simulink model "AirManagementSystem"  (R2018b)
settings: Solver=ode4  StartTime=0.0  StopTime=14400  FixedStep=dt  RelTol=1e-3
values from neighbouring files (symbols this model uses):
  AirSourceMode = 2    [run_sim.m]
  dt = 0.01    [run_sim.m]    (also in sys_id_pipeline.m = mean(diff(Time_vec_full)))
  K31 = Result31.K_slope    [sys_id_pipeline.m]
  K32 = Result32.K_slope    [sys_id_pipeline.m]
  P_ref = GlobalParams.P_ref    [sys_id_pipeline.m]
  Patm = GlobalParams.Patm    [sys_id_pipeline.m]
  R_gas = GlobalParams.R    [sys_id_pipeline.m]
  T_ref = GlobalParams.T_ref    [sys_id_pipeline.m]
  Tau31 = 5    [sys_id_pipeline.m]
  Tau32 = 5    [sys_id_pipeline.m]
  Tp31 = Result31.Tp    [sys_id_pipeline.m]
  Tp32 = Result32.Tp    [sys_id_pipeline.m]
  V_vol = pi * (0.05)^2 * 5    (= 0.0392699081699)    [run_sim.m]
  X31_den = sys_X31.Denominator    [sys_id_value.m]
  X31_num = sys_X31.Numerator    [sys_id_value.m]
  X32_den = sys_X32.Denominator    [sys_id_value.m]
  X32_num = sys_X32.Numerator    [sys_id_value.m]
libraries: simulink x8
(part 2 of 2)

== matlab function AirManagementSystem/ECS Controller/Smith_MPC_Controller/Smith_MPC_Controller ==
  settings: updateMethod=DISCRETE
  data: Q31Ref input; V31 output; Q31Real input; Q32Ref input; Q32Real input; P30 input; T30 input; V32 output; K31 parameter; Tau31 parameter; K32 parameter; Tau32 parameter; P_ref parameter; T_ref parameter; R_gas parameter; Patm parameter; Tp31 parameter; Tp32 parameter; dt parameter; X31_num parameter; X31_den parameter; X32_num parameter; X32_den parameter
function [V31, V32] = Smith_MPC_Controller(Q31Ref, Q31Real, Q32Ref, Q32Real, P30, T30, K31, Tau31, K32, Tau32, P_ref, T_ref, R_gas, Patm, Tp31, Tp32, dt, X31_num, X31_den, X32_num, X32_den)
    % Smith_MPC_Controller
    %
    % 这是一个基于 Smith 预估器的 MPC 控制器，用于替换原有的 Smith-PI 方案。
    % 核心思想：
    % 1. Smith 预估器：利用内部模型消除反馈回路中的纯滞后，使 MPC 面对一个"无滞后"的虚拟对象。
    % 2. MPC 控制：利用过程模型预测未来轨迹，在处理约束(0-100%)的前提下最小化跟踪误差。
    % 3. 测量滞后补偿：通过比较实际测量值与延时模型输出，估算当前扰动并修正 MPC 的状态估计。
    %
    % 适用性：
    % - Q31 (过阻尼): MPC 通过预测未来，能更果断地给出控制量，克服大惯性。
    % - Q32 (欠阻尼): MPC 的代价函数包含控制增量惩罚 (R_weight)，能有效抑制震荡。

    % === 1. 状态记忆区 ===
    persistent model_31 model_32            % 快速模型状态 [x1; x2; x3]
    persistent delay_buffer_31 delay_buffer_32 % 延时缓冲区
    persistent head_31 head_32              % 缓冲区指针
    persistent u_prev_31 u_prev_32          % 上一时刻控制量
    persistent first_run                    % 初始化标志
    
    MAX_BUF = 1000;

    if isempty(first_run)
        model_31 = [0;0;0]; model_32 = [0;0;0];
        delay_buffer_31 = zeros(MAX_BUF, 1);
        delay_buffer_32 = zeros(MAX_BUF, 1);
        head_31 = 1; head_32 = 1;
        u_prev_31 = 0; u_prev_32 = 0;
        first_run = 0;
    end

    % === 2. 全局参数与 MPC 配置 ===
    % 计算流量工况系数 (增益调度)
    Ratio = CalculateFlowRatio(P30, T30, P_ref, T_ref, R_gas, Patm);

    % MPC 调参指南：
    % N_p (预测时域): 看得越远越稳，但计算量大。过阻尼系统需要较长 N_p。
    % N_c (控制时域): 自由度。通常取 N_p 的 10%-20%。
    % lambda (控制权重): 越大系统越柔和（抗震荡），越小响应越快（抗惯性）。
    
    % --- 通道 31 配置 (过阻尼) ---
    % 策略：较小的 lambda 允许较大的动作来克服惯性/摩擦
    MPC_31.Np = 200;        % 预测 15 步
    MPC_31.Nc = 40;         % 控制 3 步变化
    MPC_31.lambda = 5;   % 权重较小，追求快速响应
    
    % --- 通道 32 配置 (欠阻尼) ---
    % 策略：较大的 lambda 抑制控制量的剧烈变化，防止激发震荡
    MPC_32.Np = 200;        % 预测更远，捕捉震荡趋势
    MPC_32.Nc = 40; 
    MPC_32.lambda = 50;   % 权重较大，强行增加阻尼效果

    % ==========================================================
    %       通道 31 控制回路 (MPC + Smith)
    % ==========================================================
    
    % 1. 获取离散化状态空间模型 (A, B, C)
    % 注意：将 Ratio 应用于 B 矩阵，使模型增益匹配当前物理工况
    [A31, B31, C31] = GetStateSpace(X31_num, X31_den, K31, Ratio, Tp31, dt);
    
    % 2. Smith 快速模型更新 (无滞后估计)
    % 计算假如没有滞后，当前系统应该在哪
    [model_31, Y_fast_31] = UpdateStateModel(model_31, u_prev_31, A31, B31, C31);
    
    % 3. 延时模型更新 (历史数据回放)
    [delay_buffer_31, head_31, Y_delayed_31] = UpdateDelayBuffer(delay_buffer_31, head_31, Y_fast_31, Tau31, dt, MAX_BUF);
    
    % 4. 测量滞后补偿 / 扰动估算
    % 真实值与模型值的差异，被认为是"扰动"(dist_est)
    dist_est_31 = Q31Real - Y_delayed_31;
    
    % 5. 构造 MPC 反馈状态
    % 修正后的输出 = 无滞后模型值 + 当前扰动
    % MPC 认为它在控制这个"当前"值，从而忽略了滞后
    y_feedback_31 = Y_fast_31 + dist_est_31;
    
    % 6. MPC 求解
    % 计算最优控制增量 du
    du_31 = SolveMPC(A31, B31, C31, MPC_31, model_31, y_feedback_31, Q31Ref, u_prev_31);
    
    % 7. 输出计算与限幅
    u_raw_31 = u_prev_31 + du_31;
    u_raw_31 = max(0, min(100, u_raw_31));
    
    % 8. (可选) 保留死区补偿作为最后一道防线
    % MPC 虽然能处理部分非线性，但物理阀门的静摩擦最好显式补偿
    V31 = InverseDeadzoneComp(u_raw_31, u_prev_31, 1.4, Q31Ref - y_feedback_31);
    u_prev_31 = V31;

    % ==========================================================
    %       通道 32 控制回路 (MPC + Smith)
    % ==========================================================
    
    [A32, B32, C32] = GetStateSpace(X32_num, X32_den, K32, Ratio, Tp32, dt);
    
    [model_32, Y_fast_32] = UpdateStateModel(model_32, u_prev_32, A32, B32, C32);
    [delay_buffer_32, head_32, Y_delayed_32] = UpdateDelayBuffer(delay_buffer_32, head_32, Y_fast_32, Tau32, dt, MAX_BUF);
    
    dist_est_32 = Q32Real - Y_delayed_32;
    y_feedback_32 = Y_fast_32 + dist_est_32;
    
    du_32 = SolveMPC(A32, B32, C32, MPC_32, model_32, y_feedback_32, Q32Ref, u_prev_32);
    
    u_raw_32 = u_prev_32 + du_32;
    u_raw_32 = max(0, min(100, u_raw_32));
    
    V32 = InverseDeadzoneComp(u_raw_32, u_prev_32, 0.5, Q32Ref - y_feedback_32);
    u_prev_32 = V32;

end

%% === 核心模块: MPC 求解器 (解析解法) ===
% 这是一个轻量级的无约束 MPC 求解器，通过饱和截断处理约束。
% 求解目标函数: J = sum((Y - Ref)^2) + lambda * sum(dU^2)
function du_opt = SolveMPC(A, B, C, Config, x_current, y_corrected, Ref, u_last)
    Np = Config.Np;
    Nc = Config.Nc;
    lambda = Config.lambda;
    
    % 1. 预计算预测矩阵 (Phi 和 Gamma)
    % Y = Phi * x0 + Gamma * dU
    % 注意：为了效率，这些矩阵在定常系统中可以离线计算。
    % 但由于我们有 Ratio 增益调度，B 矩阵是变的，所以必须实时计算。
    
    n = size(A, 1); % 状态维数
    Phi = zeros(Np, n);
    Gamma = zeros(Np, Nc);
    
    % 构建 Phi (自由响应部分)
    A_pow = eye(n);
    for i = 1:Np
        A_pow = A_pow * A;
        Phi(i, :) = C * A_pow;
    end
    
    % 构建 Gamma (受迫响应部分)
    % 这是一个下三角Toeplitz矩阵的变体，处理控制增量
    % 这种 formulation 基于 dU 模型 (积分型 MPC)，本身具有无静差特性
    
    % 这里的状态空间是基于物理状态 x 的。为了实现无静差，
    % 我们通常使用增量式 MPC 形式，或者在外部处理扰动（我们已经通过 Smith 做了）。
    % 在 Smith 架构下，我们只要让 y 追踪 Ref 即可。
    % 这里简化处理：假设 dU 在 Nc 步后为 0。
    
    % 临时计算阶跃响应系数 h
    h = zeros(Np, 1);
    AB_pow = B;
    for i = 1:Np
        h(i) = C * AB_pow;
        AB_pow = A * AB_pow + B; % 累积效果 (如果是位置式)
        % 修正：对于常规状态空间 x(k+1) = Ax + Bu, 
        % 阶跃响应 h(i) = C * (sum(A^(j-1)*B))
    end
    
    % 由于直接构造增量形式较复杂，这里采用简化的 DMC (Dynamic Matrix Control) 思路
    % 利用上面计算的阶跃响应 h 来填充 Gamma
    % Gamma 矩阵:
    % [h1   0    0 ]
    % [h2   h1   0 ]
    % [h3   h2   h1]
    
    % 重新计算阶跃响应序列 (Step Response)
    step_resp = zeros(Np, 1);
    x_tmp = zeros(n, 1);
    u_step = 1;
    for i = 1:Np
        x_tmp = A * x_tmp + B * u_step;
        step_resp(i) = C * x_tmp;
    end
    
    for i = 1:Np
        for j = 1:Nc
            if (i >= j)
                Gamma(i, j) = step_resp(i - j + 1);
            end
        end
    end
    
    % 2. 预测当前的自由响应 (Free Response)
    % 也就是假设未来 dU 全为 0，系统会怎么走
    % 这里的起点是 x_current。但在 Smith 结构中，我们有测量修正。
    % 修正量 = y_corrected - (C * x_current)
    % 我们把这个常数偏差加到自由响应上。
    
    dist = y_corrected - (C * x_current);
    
    % 自由响应预测
    Y_free = zeros(Np, 1);
    x_pred = x_current;
    u_curr = u_last; % 假设控制量保持不变
    for i = 1:Np
        x_pred = A * x_pred + B * u_curr;
        Y_free(i) = C * x_pred + dist; % 加上扰动估计
    end
    
    % 3. 构造误差向量
    E = Ref * ones(Np, 1) - Y_free;
    
    % 4. 求解最优 dU
    % 解析解: dU = (Gamma' * Gamma + lambda * I)^-1 * Gamma' * E
    H = Gamma' * Gamma + lambda * eye(Nc);
    f = -Gamma' * E;
    
    % 如果矩阵很小(Nc=3)，直接求逆很快
    dU_seq = -H \ f;
    
    % 取第一个控制增量
    du_opt = dU_seq(1);
    
    % 简单的饱和处理 (防积分饱和的一种形式)
    % 检查应用 du_opt 后是否超出 0-100
    if (u_last + du_opt) > 100
        du_opt = 100 - u_last;
    elseif (u_last + du_opt) < 0
        du_opt = 0 - u_last;
    end
end

%% === 辅助模块: 模型转换 ===
% 将传递函数参数转换为离散状态空间 A, B, C
function [A, B, C] = GetStateSpace(num, den, K, Ratio, Tp, Ts)
    % 阀门二阶: num / (s^2 + den(2)s + den(3)) -> 实际上 den 可能是 [1 2*zw*wn wn^2]
    % 这里沿用原代码逻辑：acc = K_valve * u - zw * x2 - wn2 * x1
    % 原代码系数映射: wn2 = den(3), zw = den(2), K_valve = num
    
    wn2 = den(3);
    zw = den(2);
    K_valve = num;
    K_total = K * Ratio; % 增益调度
    
    % 连续时间矩阵 (Ac, Bc)
    % 状态: [x1(阀位), x2(阀速), x3(流量)]
    % dx1 = x2
    % dx2 = -wn2*x1 - zw*x2 + K_valve*u
    % dx3 = (K_total*x1 - x3)/Tp
    
    % 离散化 (Euler 近似，与原代码一致，保持物理意义)
    % x1(k+1) = x1(k) + Ts*x2(k)
    % x2(k+1) = x2(k) - Ts*wn2*x1(k) - Ts*zw*x2(k) + Ts*K_valve*u(k)
    % x3(k+1) = x3(k) + (Ts*K_total/Tp)*x1(k) - (Ts/Tp)*x3(k)
    
    Tp = max(Tp, 0.1); % 保护
    
    A = [1,          Ts,               0;
         -Ts*wn2,    1 - Ts*zw,        0;
         Ts*K_total/Tp, 0,             1 - Ts/Tp];
         
    B = [0;
         Ts * K_valve;
         0];
         
    C = [0, 0, 1];
end

%% === 辅助模块: 模型状态更新 ===
function [state_new, y_out] = UpdateStateModel(state, u, A, B, C)
    state_new = A * state + B * u;
    y_out = C * state_new;
end

%% === 辅助模块: 延时队列 ===
function [buffer, head_idx, y_delayed] = UpdateDelayBuffer(buffer, head, y_in, Tau, Ts, MAX_BUF)
    delay_steps = round(Tau / Ts);
    delay_steps = max(1, min(delay_steps, MAX_BUF - 1));
    buffer(head) = y_in;
    read_idx = head - delay_steps;
    if read_idx < 1, read_idx = read_idx + MAX_BUF; end
    y_delayed = buffer(read_idx);
    head_idx = head + 1;
    if head_idx > MAX_BUF, head_idx = 1; end
end

%% === 辅助模块: 物理死区补偿 ===
function u_final = InverseDeadzoneComp(u_cmd, u_last, gap, error)
    % 简化的死区补偿，仅在需要动作时叠加脉冲
    delta = u_cmd - u_last;
    threshold = 0.05; % 动作死区
    
    if abs(delta) > threshold
        if delta > 0
            u_final = u_cmd + gap;
        else
            u_final = u_cmd - gap;
        end
    else
        u_final = u_cmd; % 如果 MPC 认为不需要大动，就不加 Gap
    end
end

%% === 辅助模块: 工况计算 ===
function Ratio = CalculateFlowRatio(P30, T30, P_ref, T_ref, R_gas, Patm)
    Tk_dyn = T30 + 273.15; delta_P_dyn = P30 - Patm;
    if delta_P_dyn < 0, delta_P_dyn = 0; end
    Term_Dyn = sqrt((P30 * 1000 * delta_P_dyn * 1000) / (R_gas * Tk_dyn));
    Tk_ref = T_ref + 273.15; delta_P_ref = P_ref - Patm;
    if delta_P_ref < 0, delta_P_ref = 0; end
    Term_Ref = sqrt((P_ref * 1000 * delta_P_ref * 1000) / (R_gas * Tk_ref));
    if Term_Ref < 1e-6, Ratio = 1; else, Ratio = max(Term_Dyn / Term_Ref, 0.05); end
end

== matlab function AirManagementSystem/Engine Bleed Air System/Precooler/BleedAirSource ==
  data: clockTime input; P_comp output; T_comp output; P_fan output; T_fan output; AirSourceMode input
function [P_comp, T_comp, P_fan, T_fan] = BleedAirSource(clockTime, AirSourceMode)
    % =========================================================================
    % 飞机环境与引气参数模拟源
    %
    % 输入: 
    %   clockTime : 仿真时间 [s]
    %   AirSourceMode   : 仿真模式选择
    %                       1 = 动态任务剖面 (Dynamic Mission Profile)
    %                       2 = 静态设计点 (Static Design Point)
    %                       3 = 静态设计点 + 正弦波动 (Static + Sine Wave)
    % 输出: 
    %   P_comp: 热路引气压力 [kPa]
    %   T_comp: 热路引气温度 [degC]
    %   P_fan : 冷路风扇压力 [kPa]
    %   T_fan : 冷路风扇温度 [degC]
    % =========================================================================

    if AirSourceMode == 1
        % =================================================================
        % 模式 1: 动态飞行任务剖面 (随时间变化)
        % =================================================================
        
        % 1. 定义飞行剖面节点 [时间(s), 高度(m)]
        t_points = [0,    2000, 4000, 6000,  8000,  10000, 12000, 14000];
        h_points = [0,    7620, 7620, 12192, 12192, 9144,  9144, 0];
        
        t_safe = max(min(clockTime, 14000), 0); % 限制时间范围
        
        % 2. 计算当前高度 (线性插值)
        Alt = interp1(t_points, h_points, t_safe, 'linear');
        
        % 3. 计算国际标准大气 (ISA)
        % 温度递减率: -6.5 C/km
        % 海平面: 15 C, 101.325 kPa
        T_amb_C = 15 - 0.0065 * Alt;
        T_amb_K = T_amb_C + 273.15;
        % 压力高度公式 (对流层)
        P_amb_kPa = 101.325 * (1 - 2.25577e-5 * Alt)^5.2559;
        
        % 4. 发动机参数解算
        Gamma = 1.4;
        
        % --- 冷路 (Fan) ---
        FPR = 1.6; % 风扇压比
        P_fan = P_amb_kPa * FPR;
        % 绝热压缩温升
        T_fan_K = T_amb_K * (FPR^((Gamma-1)/Gamma));
        T_fan = T_fan_K - 273.15;        % 输出摄氏度
        
        % --- 热路 (Compressor) ---
        CPR = 12; % 压气机压比
        eff = 0.85; % 绝热效率
        P_comp = P_amb_kPa * CPR;
        % 压气机出口温度计算
        T_comp_K = T_amb_K * (1 + (CPR^((Gamma-1)/Gamma) - 1) / eff);
        T_comp = T_comp_K - 273.15; % 输出摄氏度
        
    elseif AirSourceMode == 2
        % =================================================================
        % 模式 2: 静态设计点 (常值)
        % 适用于PID参数整定或稳态特性研究
        % =================================================================
        
        % 热路设定 (典型高压引气)
        P_comp = 600;   % [kPa]
        T_comp = 280;   % [degC]
        
        % 冷路设定 (典型地面或低空风扇出口)
        P_fan  = 110;   % [kPa]
        T_fan  = 30;    % [degC]

    elseif AirSourceMode == 3
        % =================================================================
        % 模式 3: 静态设计点 + 正弦波动干扰
        % 适用于测试控制系统的抗干扰能力和动态调节性能
        % =================================================================

        % --- 基础静态值 (与模式2相同) ---
        Base_P_comp = 600;
        Base_T_comp = 280;
        Base_P_fan  = 110;
        Base_T_fan  = 30;

        % --- 波动参数设置 ---
        % 频率 Hz (0.01 Hz = 100秒一个周期)
        Freq_P = 0.01; 
        Freq_T = 0.005; % 温度变化通常比压力慢，设为更低频率

        % 振幅 (波动的大小)
        Amp_P_comp = 20;  % 压力波动 +/- 50 kPa
        Amp_T_comp = 5;  % 温度波动 +/- 5 degC
        Amp_P_fan  = 5;  % 风扇压力波动较小
        Amp_T_fan  = 5;   

        % --- 计算波动值 ---
        % 公式: Base + Amplitude * sin(2 * pi * f * t)
        P_comp = Base_P_comp + Amp_P_comp * sin(2 * pi * Freq_P * clockTime);
        T_comp = Base_T_comp + Amp_T_comp * sin(2 * pi * Freq_T * clockTime);
        
        P_fan  = Base_P_fan  + Amp_P_fan  * sin(2 * pi * Freq_P * clockTime);
        T_fan  = Base_T_fan  + Amp_T_fan  * sin(2 * pi * Freq_T * clockTime);

    else
        % 默认防错输出
        P_comp = 101.3;
        T_comp = 15;
        P_fan = 101.3;
        T_fan = 15;
    end

end

== matlab function AirManagementSystem/EBAS Controller/L1AC Controller/PRSOV L1AC Controller ==
  data: Target input; u_cmd output; Measured input; P_L1 parameter
function u_cmd = L1_Controller(Target, Measured, P_L1)
    % =========================================================================
    % L1 Adaptive Controller (Discrete Time Implementation)
    % 
    % Inputs:
    %   Target   - 设定值 (如目标压力 480kPa 或目标温度 200C)
    %   Measured - 实际测量值
    %   Am       - 参考模型带宽 (期望的系统响应速度, >0)
    %   Gamma    - 自适应增益 (学习率, 越大收敛越快但可能震荡)
    %   Bm       - 标称控制增益 (估算的系统输入效能 B矩阵)
    %   Wc       - L1滤波器截止频率 (决定了控制器的频带宽度)
    %
    % Output:
    %   u_cmd    - 控制指令 (0~1)
    % =========================================================================
    
    Am = P_L1.Press.Am;
    Gamma = P_L1.Press.Gamma;
    Bm = P_L1.Press.Bm;
    Wc = P_L1.Press.Wc;

    % --- 状态记忆 ---
    persistent x_hat      % 状态观测值 (Predictor State)
    persistent sigma_hat  % 扰动/不确定性估计值 (Adaptive Estimate)
    persistent u_filter   % 经过滤波后的控制量 (Filtered Control)
    
    % --- 采样时间 ---
    % 必须与 Simulink Solver 的 Fixed-step size 保持一致
    dt = 0.01; 
    
    % --- 初始化 ---
    if isempty(x_hat)
        x_hat = Measured; % 初始观测值跟随测量值
        sigma_hat = 0;
        u_filter = 0;     % 假设初始阀门关闭或处于某个中间值
    end
    
    % =====================================================================
    % 1. 状态预测器 (State Predictor)
    %    理论模型: x_dot_hat = -Am * x_hat + Bm * u + sigma_hat
    %    x_hat 试图追踪真实的 Measured 值，两者的差异驱动自适应律
    % =====================================================================
    % 使用上一时刻的控制量 u_filter 进行预测
    x_hat_dot = -Am * x_hat + Bm * u_filter + sigma_hat;
    
    % 欧拉积分更新预测状态
    x_hat_next = x_hat + x_hat_dot * dt;
    
    % =====================================================================
    % 2. 误差计算 (Prediction Error)
    %    x_tilde = x_hat - x_real
    % =====================================================================
    x_tilde = x_hat - Measured;
    
    % =====================================================================
    % 3. 自适应律 (Adaptation Law)
    %    sigma_dot_hat = -Gamma * x_tilde
    %    基于 Lyapunov 稳定性推导，用于快速估计总扰动 sigma
    % =====================================================================
    sigma_dot = -Gamma * x_tilde;
    
    % 更新扰动估计
    sigma_hat_next = sigma_hat + sigma_dot * dt;
    
    % =====================================================================
    % 4. 控制律计算 (Control Law)
    %    目标: 消除扰动 sigma 并跟踪参考信号 Target
    %    u_raw = (Am * Target - sigma_hat) / Bm
    %    (这里假设我们希望闭环系统行为像 dx/dt = -Am*x + Am*Target)
    % =====================================================================
    u_raw = (Am * Target - sigma_hat_next) / Bm;
    
    % =====================================================================
    % 5. 低通滤波器 (Low-Pass Filter) - L1 控制器的关键特征
    %    C(s) = Wc / (s + Wc)
    %    过滤掉高频自适应噪声，仅让低频有效控制信号通过
    % =====================================================================
    u_dot = -Wc * u_filter + Wc * u_raw;
    u_filter_next = u_filter + u_dot * dt;
    
    % =====================================================================
    % 6. 输出限幅与状态更新
    % =====================================================================
    % 物理执行机构限制 (0 ~ 1)
    u_cmd = max(min(u_filter_next, 1), 0);
    
    % 更新 Persistent 变量供下一次计算使用
    x_hat = x_hat_next;
    sigma_hat = sigma_hat_next;
    
    % 注意：这里使用限幅后的 u_cmd 更新 u_filter，
    % 可以在一定程度上防止积分器(滤波器)饱和 (Anti-windup 效应)
    u_filter = u_cmd; 
end

== matlab function AirManagementSystem/EBAS Controller/L1AC Controller/FAV L1AC Controller ==
  data: Target input; u_cmd output; Measured input; P_L1 parameter
function u_cmd = L1_Controller(Target, Measured, P_L1)
    % =========================================================================
    % L1 Adaptive Controller (Discrete Time Implementation)
    % 
    % Inputs:
    %   Target   - 设定值 (如目标压力 480kPa 或目标温度 200C)
    %   Measured - 实际测量值
    %   Am       - 参考模型带宽 (期望的系统响应速度, >0)
    %   Gamma    - 自适应增益 (学习率, 越大收敛越快但可能震荡)
    %   Bm       - 标称控制增益 (估算的系统输入效能 B矩阵)
    %   Wc       - L1滤波器截止频率 (决定了控制器的频带宽度)
    %
    % Output:
    %   u_cmd    - 控制指令 (0~1)
    % =========================================================================
    
    Am = P_L1.Temp.Am;
    Gamma = P_L1.Temp.Gamma;
    Bm = P_L1.Temp.Bm;
    Wc = P_L1.Temp.Wc;

    % --- 状态记忆 ---
    persistent x_hat      % 状态观测值 (Predictor State)
    persistent sigma_hat  % 扰动/不确定性估计值 (Adaptive Estimate)
    persistent u_filter   % 经过滤波后的控制量 (Filtered Control)
    
    % --- 采样时间 ---
    % 必须与 Simulink Solver 的 Fixed-step size 保持一致
    dt = 0.01; 
    
    % --- 初始化 ---
    if isempty(x_hat)
        x_hat = Measured; % 初始观测值跟随测量值
        sigma_hat = 0;
        u_filter = 0;     % 假设初始阀门关闭或处于某个中间值
    end
    
    % =====================================================================
    % 1. 状态预测器 (State Predictor)
    %    理论模型: x_dot_hat = -Am * x_hat + Bm * u + sigma_hat
    %    x_hat 试图追踪真实的 Measured 值，两者的差异驱动自适应律
    % =====================================================================
    % 使用上一时刻的控制量 u_filter 进行预测
    x_hat_dot = -Am * x_hat + Bm * u_filter + sigma_hat;
    
    % 欧拉积分更新预测状态
    x_hat_next = x_hat + x_hat_dot * dt;
    
    % =====================================================================
    % 2. 误差计算 (Prediction Error)
    %    x_tilde = x_hat - x_real
    % =====================================================================
    x_tilde = x_hat - Measured;
    
    % =====================================================================
    % 3. 自适应律 (Adaptation Law)
    %    sigma_dot_hat = -Gamma * x_tilde
    %    基于 Lyapunov 稳定性推导，用于快速估计总扰动 sigma
    % =====================================================================
    sigma_dot = -Gamma * x_tilde;
    
    % 更新扰动估计
    sigma_hat_next = sigma_hat + sigma_dot * dt;
    
    % =====================================================================
    % 4. 控制律计算 (Control Law)
    %    目标: 消除扰动 sigma 并跟踪参考信号 Target
    %    u_raw = (Am * Target - sigma_hat) / Bm
    %    (这里假设我们希望闭环系统行为像 dx/dt = -Am*x + Am*Target)
    % =====================================================================
    u_raw = (Am * Target - sigma_hat_next) / Bm;
    
    % =====================================================================
    % 5. 低通滤波器 (Low-Pass Filter) - L1 控制器的关键特征
    %    C(s) = Wc / (s + Wc)
    %    过滤掉高频自适应噪声，仅让低频有效控制信号通过
    % =====================================================================
    u_dot = -Wc * u_filter + Wc * u_raw;
    u_filter_next = u_filter + u_dot * dt;
    
    % =====================================================================
    % 6. 输出限幅与状态更新
    % =====================================================================
    % 物理执行机构限制 (0 ~ 1)
    u_cmd = max(min(u_filter_next, 1), 0);
    
    % 更新 Persistent 变量供下一次计算使用
    x_hat = x_hat_next;
    sigma_hat = sigma_hat_next;
    
    % 注意：这里使用限幅后的 u_cmd 更新 u_filter，
    % 可以在一定程度上防止积分器(滤波器)饱和 (Anti-windup 效应)
    u_filter = u_cmd; 
end

== matlab function AirManagementSystem/Engine Bleed Air System/FAV Actuator ==
  data: cmd_FAV_mA input; theta_FAV output; dt parameter
function theta_FAV = FAV_Actuator(cmd_FAV_mA, dt)
    % =========================================================================
    % FAV 执行机构模型 
    % 
    % 功能: 将电流转换为阀门角度，包含磁滞和动态特性
    % 输入: 
    %   cmd_PRSOV_mA - 控制电流 (0-400mA)
    % 输出: 
    %   theta_PRSOV - 阀门物理角度 (0-90度)
    % =========================================================================

    % 记忆上一次的状态
    persistent Prev_Hys_Angle Prev_Angle is_initialized
    
    % --- 1. 动态初始化 ---
    % 如果是第一次运行，根据当前电流计算初始角度
    if isempty(is_initialized)
        I_start = max(0, min(cmd_FAV_mA, 350));
        
        % 定义基础特性数据
        I_data = [0, 120.0000, 134.3750, 148.7500, 163.1250, 177.5000, ...
              206.2500, 235.0000, 263.7500, 292.5000, 321.2500, 350.0000];
        A_rise_data = [0, 0, 3, 7, 15, 25, 45, 62, 75, 85, 89, 90]; 
        A_fall_data = [0, 0, 10, 25, 40, 55, 75, 85, 89, 90, 90, 90];
        
        % 初始角度
        Prev_Hys_Angle = 0;
        Prev_Angle = Prev_Hys_Angle;
        is_initialized = true;
    end
    
    % --- 2. 输入限幅 ---
    I_safe = max(0, min(cmd_FAV_mA, 350));
    
    % --- 3. 磁滞包络线计算 ---
    I_ref = [0, 120.0000, 134.3750, 148.7500, 163.1250, 177.5000, ...
              206.2500, 235.0000, 263.7500, 292.5000, 321.2500, 350.0000];
    A_rise = [0, 0, 3, 7, 15, 25, 45, 62, 75, 85, 89, 90]; 
    A_fall = [0, 0, 10, 25, 40, 55, 75, 85, 89, 90, 90, 90];
    
    % 计算当前电流对应的上下限
    Limit_Low  = interp1(I_ref, A_rise, I_safe, 'linear', 'extrap');
    Limit_High = interp1(I_ref, A_fall, I_safe, 'linear', 'extrap');
    
    % 限制范围在 0 到 90 度
    Limit_Low  = max(0, min(90, Limit_Low));
    Limit_High = max(0, min(90, Limit_High));
    
    % --- 4. 磁滞逻辑实现 ---
    % 如果电流变化没超过包络线，角度保持不变
    Target_Angle = max(Limit_Low, min(Limit_High, Prev_Hys_Angle));
    Prev_Hys_Angle = Target_Angle;
    
    % --- 5. 惯性环节 (一阶响应) ---
    Tau = 0.1; % 时间常数
    % 使用输入的 dt 计算新角度
    Angle_new = Prev_Angle + (Target_Angle - Prev_Angle) * (dt / (Tau + dt));
    
    % 更新并输出结果
    Prev_Angle = Angle_new;
    theta_FAV = Angle_new;
end

== matlab function AirManagementSystem/Reference Generator/GetRefValue_THQ ==
  data: clockTime input; thMap input; hQ31Map input; hQ32Map input; Q31RefthQ output; Q32RefthQ output
function [Q31RefthQ, Q32RefthQ] = getRefValue_THQ(clockTime, thMap, hQ31Map, hQ32Map)
    elapsedTime = max(min(clockTime, max(thMap(:,1))), min(thMap(:,1)));
    
    % 排序 + 去重（按高度第一列）
    thMap   = sortrows(thMap, 1);    [~, idx_th] = unique(thMap(:,1), 'stable'); thMap = thMap(idx_th, :);
    hQ31Map = sortrows(hQ31Map, 1);  [~, idx31] = unique(hQ31Map(:,1), 'stable'); hQ31Map = hQ31Map(idx31, :);
    hQ32Map = sortrows(hQ32Map, 1);  [~, idx32] = unique(hQ32Map(:,1), 'stable'); hQ32Map = hQ32Map(idx32, :);

    % 计算当前高度（时间 → 高度）
    currentHeight = interp1(thMap(:,1), thMap(:,2), elapsedTime, 'linear', 'extrap');

    % 获取各流量的最小和最大高度
    minHeight_Q31 = min(hQ31Map(:,1)); maxHeight_Q31 = max(hQ31Map(:,1));
    minHeight_Q32 = min(hQ32Map(:,1)); maxHeight_Q32 = max(hQ32Map(:,1));

    % 限制 currentHeight 在各自的高度范围内
    height_Q31 = min(max(currentHeight, minHeight_Q31), maxHeight_Q31);
    height_Q32 = min(max(currentHeight, minHeight_Q32), maxHeight_Q32);

    % 计算各个流量值（高度 → 流量）
    Q31RefthQ = interp1(hQ31Map(:,1), hQ31Map(:,2), height_Q31, 'linear', 'extrap');
    Q32RefthQ = interp1(hQ32Map(:,1), hQ32Map(:,2), height_Q32, 'linear', 'extrap');
end

== matlab function AirManagementSystem/Engine Bleed Air System/PRSOV Actuator ==
  data: cmd_PRSOV_mA input; theta_PRSOV output; dt parameter
function theta_PRSOV = PRSOV_Actuator(cmd_PRSOV_mA, dt)
    % =========================================================================
    % PRSOV 执行机构模型 
    % 
    % 功能: 将电流转换为阀门角度，包含磁滞和动态特性
    % 输入: 
    %   cmd_PRSOV_mA - 控制电流 (0-400mA)
    % 输出: 
    %   theta_PRSOV - 阀门物理角度 (0-90度)
    % =========================================================================

    % 记忆上一次的状态
    persistent Prev_Hys_Angle Prev_Angle is_initialized
    
    % --- 1. 动态初始化 ---
    % 如果是第一次运行，根据当前电流计算初始角度
    if isempty(is_initialized)
        I_start = max(0, min(cmd_PRSOV_mA, 400));
        
        % 定义基础特性数据
        I_data = [0, 120.0, 137.5, 155.0, 172.5, 190.0, 225.0, 260.0, 295.0, 330.0, 365.0, 400.0];
        A_rise_data = [0, 0, 3, 7, 15, 25, 45, 62, 75, 85, 89, 90]; 
        A_fall_data = [0, 0, 10, 25, 40, 55, 75, 85, 89, 90, 90, 90];
        
        % 初始角度
        Prev_Hys_Angle = 0;
        Prev_Angle = Prev_Hys_Angle;
        is_initialized = true;
    end
    
    % --- 2. 输入限幅 ---
    I_safe = max(0, min(cmd_PRSOV_mA, 400));
    
    % --- 3. 磁滞包络线计算 ---
    I_ref = [0, 120.0, 137.5, 155.0, 172.5, 190.0, 225.0, 260.0, 295.0, 330.0, 365.0, 400.0];
    A_rise = [0, 0, 3, 7, 15, 25, 45, 62, 75, 85, 89, 90]; 
    A_fall = [0, 0, 10, 25, 40, 55, 75, 85, 89, 90, 90, 90];
    
    % 计算当前电流对应的上下限
    Limit_Low  = interp1(I_ref, A_rise, I_safe, 'linear', 'extrap');
    Limit_High = interp1(I_ref, A_fall, I_safe, 'linear', 'extrap');
    
    % 限制范围在 0 到 90 度
    Limit_Low  = max(0, min(90, Limit_Low));
    Limit_High = max(0, min(90, Limit_High));
    
    % --- 4. 磁滞逻辑实现 ---
    % 如果电流变化没超过包络线，角度保持不变
    Target_Angle = max(Limit_Low, min(Limit_High, Prev_Hys_Angle));
    Prev_Hys_Angle = Target_Angle;
    
    % --- 5. 惯性环节 (一阶响应) ---
    Tau = 0.1; % 时间常数
    % 使用输入的 dt 计算新角度
    Angle_new = Prev_Angle + (Target_Angle - Prev_Angle) * (dt / (Tau + dt));
    
    % 更新并输出结果
    Prev_Angle = Angle_new;
    theta_PRSOV = Angle_new;
end

== matlab function AirManagementSystem/ECS Controller/Smith_iLQR_Integral_Controller/Smith_iLQR_Integral_Controller ==
  settings: updateMethod=DISCRETE
  data: Q31Ref input; V31 output; Q31Real input; Q32Ref input; Q32Real input; P30 input; T30 input; V32 output; K31 parameter; Tau31 parameter; K32 parameter; Tau32 parameter; P_ref parameter; T_ref parameter; R_gas parameter; Patm parameter; X31_num parameter; X31_den parameter; X32_num parameter; Tp31 parameter; X32_den parameter; Tp32 parameter; dt parameter
function [V31, V32] = Smith_iLQR_Integral_Controller(Q31Ref, Q31Real, Q32Ref, Q32Real, P30, T30, K31, Tau31, K32, Tau32, P_ref, T_ref, R_gas, Patm, X31_num, X31_den, X32_num, Tp31, X32_den, Tp32, dt)
    % Smith_iLQR_Integral_Controller
    %
    % 更新日志:
    % - [New] Q32 增加了自适应 R 权重 (Adaptive R) 策略。
    %   原理：大误差时关闭平滑惩罚(R=0)以求快；小误差时开启强平滑惩罚(R=20)以求稳。
    %
    % 核心思路:
    % 1. Smith 预估 + 积分型 iLQR (消除稳态误差)
    % 2. 状态扩充：x = [阀位; 阀速; 流量; 误差积分]

    persistent model_31 model_32            
    persistent delay_buffer_31 delay_buffer_32 
    persistent head_31 head_32              
    persistent u_prev_31 u_prev_32          
    persistent u_opt_guess_31 u_opt_guess_32 
    persistent x_int_31 x_int_32
    persistent first_run

    MAX_BUF = 1000; 
    HORIZON = 20; 

    if isempty(first_run)
        model_31 = [0;0;0]; model_32 = [0;0;0];
        x_int_31 = 0; x_int_32 = 0;
        
        delay_buffer_31 = zeros(MAX_BUF, 1);
        delay_buffer_32 = zeros(MAX_BUF, 1);
        head_31 = 1; head_32 = 1;
        u_prev_31 = 0; u_prev_32 = 0;
        u_opt_guess_31 = zeros(HORIZON, 1); 
        u_opt_guess_32 = zeros(HORIZON, 1);
        first_run = 0;
    end

    Ratio = CalculateFlowRatio(P30, T30, P_ref, T_ref, R_gas, Patm);

    % === 权重配置 ===
    
    % 通道 31 (过阻尼): 保持原样
    Weights_31.Q = 0.7;
    Weights_31.Ki = 2.4;
    Weights_31.R = 0.1;
    
    % 通道 32 (欠阻尼): R 值将在后续代码中根据误差动态重写
    Weights_32.Q = 1.8;   
    Weights_32.Ki = 6.3;
    Weights_32.R = 0.0; % 初始值，会被覆盖

    % 稳态死区
    Err_Band_31 = 0.2; 
    Err_Band_32 = 0.2;

    % ==========================================================
    %       通道 31 (Channel 31)
    % ==========================================================
    [A31, B31] = GetStateSpace(X31_num, X31_den, K31, Ratio, Tp31, dt);
    
    [model_31, Y_fast_31] = UpdateFastModel_StateSpace(model_31, u_prev_31, A31, B31);
    [delay_buffer_31, head_31, Y_delayed_31] = UpdateDelayBuffer(delay_buffer_31, head_31, Y_fast_31, Tau31, dt, MAX_BUF);
    
    pred_error_31 = Q31Real - Y_delayed_31;
    Target_31 = Q31Ref - pred_error_31;
    
    err_fast_31 = Target_31 - Y_fast_31;
    
    if u_prev_31 > 0 && u_prev_31 < 100
        x_int_31 = x_int_31 + err_fast_31 * dt;
    else
        if (u_prev_31 >= 100 && err_fast_31 < 0) || (u_prev_31 <= 0 && err_fast_31 > 0)
             x_int_31 = x_int_31 + err_fast_31 * dt;
        end
    end

    x0_aug_31 = [model_31; x_int_31];
    real_err_31 = Q31Ref - Q31Real;
    
    if abs(real_err_31) < Err_Band_31
        u_raw_31 = u_prev_31;
    else
        [u_raw_31, u_opt_guess_31] = Run_iLQR_Augmented(x0_aug_31, Target_31, u_prev_31, ...
                                                        A31, B31, Weights_31, u_opt_guess_31, HORIZON, dt);
    end

    Gap_31 = 1.4; 
    V31 = InverseDeadzoneComp_Soft(u_raw_31, u_prev_31, Gap_31, real_err_31, 1.5);
    u_prev_31 = V31;

    % ==========================================================
    %       通道 32 (Channel 32)
    % ==========================================================
    [A32, B32] = GetStateSpace(X32_num, X32_den, K32, Ratio, Tp32, dt);
    
    [model_32, Y_fast_32] = UpdateFastModel_StateSpace(model_32, u_prev_32, A32, B32);
    [delay_buffer_32, head_32, Y_delayed_32] = UpdateDelayBuffer(delay_buffer_32, head_32, Y_fast_32, Tau32, dt, MAX_BUF);
    
    pred_error_32 = Q32Real - Y_delayed_32;
    Target_32 = Q32Ref - pred_error_32;

    err_fast_32 = Target_32 - Y_fast_32;
    
    if u_prev_32 > 0 && u_prev_32 < 100
        x_int_32 = x_int_32 + err_fast_32 * dt;
    else
         if (u_prev_32 >= 100 && err_fast_32 < 0) || (u_prev_32 <= 0 && err_fast_32 > 0)
             x_int_32 = x_int_32 + err_fast_32 * dt;
         end
    end

    x0_aug_32 = [model_32; x_int_32];
    real_err_32 = Q32Ref - Q32Real;

    % === [新增逻辑] 32路 自适应 R 权重调整 ===
    % 策略：大误差 -> 松刹车 (R小)；小误差 -> 踩死刹车 (R大)
    Adaptive_Threshold_32 = 20; % 误差分界线 (可根据实际情况微调)
    
    if abs(real_err_32) > Adaptive_Threshold_32
        % 误差大：关闭阻尼，全速响应
        Weights_32.R = 0.00; 
    else
        % 误差小：开启强阻尼，抑制震荡
        % R = 20.0 是一个非常强的值，能有效按住阀门
        Weights_32.R = 0.035; 
    end

    % 运行优化器
    if abs(real_err_32) < Err_Band_32
        u_raw_32 = u_prev_32;
    else
        [u_raw_32, u_opt_guess_32] = Run_iLQR_Augmented(x0_aug_32, Target_32, u_prev_32, ...
                                                        A32, B32, Weights_32, u_opt_guess_32, HORIZON, dt);
    end

    Gap_32 = 0.6;
    V32 = InverseDeadzoneComp_Soft(u_raw_32, u_prev_32, Gap_32, real_err_32, 0.5);
    u_prev_32 = V32;
end

%% === 核心模块: 增广 iLQR 优化器 ===
function [u_optimal, u_guess_next] = Run_iLQR_Augmented(x0_aug, Ref, u_last, A_phys, B_phys, W, u_guess, N, dt)
    C_phys = [0, 0, 1]; 
    Aa = [A_phys, zeros(3,1); -C_phys*dt, 1];
    Ba = [B_phys; 0];

    Q_cost = W.Q;
    R_cost = W.R;
    Ki_cost = W.Ki; 
    
    alpha = 0.15; 
    max_iter = 5; 

    U = [u_guess(2:end); u_guess(end)]; 
    
    for iter = 1:max_iter
        X_traj = zeros(4, N+1); 
        X_traj(:, 1) = x0_aug;
        for k = 1:N
            x_next = Aa * X_traj(:, k) + Ba * U(k);
            x_next(4) = x_next(4) + Ref * dt;
            X_traj(:, k+1) = x_next;
        end
        
        delta_J_U = zeros(N, 1);
        lambda = zeros(4, 1); 
        u_prev_step = u_last;
        
        for k = N:-1:1
            x_curr = X_traj(:, k+1);
            y_curr = C_phys * x_curr(1:3); 
            int_curr = x_curr(4);          
            
            if k > 1, u_act = U(k); u_prev_act = U(k-1);
            else, u_act = U(k); u_prev_act = u_prev_step; end
            
            grad_x_phys = 2 * Q_cost * C_phys' * (y_curr - Ref);
            grad_x_int = 2 * Ki_cost * int_curr;
            grad_x_aug = [grad_x_phys; grad_x_int];
            
            lambda = Aa' * lambda + grad_x_aug;
            
            grad_u_smooth = 2 * R_cost * (u_act - u_prev_act);
            delta_J_U(k) = Ba' * lambda + grad_u_smooth;
        end
        
        U = U - alpha * delta_J_U;
        U = max(0, min(100, U));
    end
    u_optimal = U(1);       
    u_guess_next = U;       
end

%% === 辅助模块 ===
function [A, B] = GetStateSpace(num, den, K, Ratio, Tp, Ts)
    wn2 = den(3); zw = den(2); K_valve = num; K_total = K * Ratio;
    A = [1, Ts, 0; -wn2*Ts, 1 - zw*Ts, 0; K_total*Ts/max(Tp,0.1), 0, 1 - Ts/max(Tp,0.1)];
    B = [0; K_valve * Ts; 0];
end

function [state_new, y_out] = UpdateFastModel_StateSpace(state, u, A, B)
    state_new = A * state + B * u;
    y_out = state_new(3); 
end

function [buffer, head_idx, y_delayed] = UpdateDelayBuffer(buffer, head, y_in, Tau, Ts, MAX_BUF)
    delay_steps = round(Tau / Ts);
    delay_steps = max(1, min(delay_steps, MAX_BUF - 1));
    buffer(head) = y_in;
    read_idx = head - delay_steps;
    if read_idx < 1, read_idx = read_idx + MAX_BUF; end
    y_delayed = buffer(read_idx);
    head_idx = head + 1;
    if head_idx > MAX_BUF, head_idx = 1; end
end

function Ratio = CalculateFlowRatio(P30, T30, P_ref, T_ref, R_gas, Patm)
    Tk_dyn = T30 + 273.15; delta_P_dyn = P30 - Patm;
    if delta_P_dyn < 0, delta_P_dyn = 0; end
    Term_Dyn = sqrt((P30 * 1000 * delta_P_dyn * 1000) / (R_gas * Tk_dyn));
    Tk_ref = T_ref + 273.15; delta_P_ref = P_ref - Patm;
    if delta_P_ref < 0, delta_P_ref = 0; end
    Term_Ref = sqrt((P_ref * 1000 * delta_P_ref * 1000) / (R_gas * Tk_ref));
    if Term_Ref < 1e-6, Ratio = 1; else, Ratio = max(Term_Dyn / Term_Ref, 0.05); end
end

function u_final = InverseDeadzoneComp_Soft(u_cmd, u_last, gap, error, err_threshold)
    delta = u_cmd - u_last;
    alpha = min(abs(error) / err_threshold, 1.0);
    real_gap = gap * alpha;
    Noise_Threshold = 0.02; 
    if abs(delta) > Noise_Threshold 
        if delta > 0, u_final = u_cmd + real_gap; else, u_final = u_cmd - real_gap; end
    else, u_final = u_last; end
    u_final = max(0, min(100, u_final));
end

== matlab function AirManagementSystem/ECS Controller/Smith_PI_Controller/Smith_PI_Controller ==
  settings: updateMethod=DISCRETE
  data: Q31Ref input; V31 output; Q31Real input; Q32Ref input; Q32Real input; P30 input; T30 input; V32 output; K31 parameter; Tau31 parameter; K32 parameter; Tau32 parameter; P_ref parameter; T_ref parameter; R_gas parameter; Patm parameter; X31_num parameter; X31_den parameter; X32_num parameter; Tp31 parameter; X32_den parameter; Tp32 parameter
function [V31, V32] = Smith_PI_Controller(Q31Ref, Q31Real, Q32Ref, Q32Real, P30, T30, K31, Tau31, K32, Tau32, P_ref, T_ref, R_gas, Patm, X31_num, X31_den, X32_num, Tp31, X32_den, Tp32)
    % Smith_PI_Controller_Optimized
    %
    % 本函数实现了一种针对双通道非线性流量控制系统的优化 Smith 预估 PI 控制策略。
    % 针对两路子系统（Q31和Q32）显著不同的动态特性（过阻尼 vs 欠阻尼）以及共同存在的
    % 执行器死区（Actuator Deadzone）和纯滞后（Pure Time Delay）问题，
    % 采用了差异化的控制律设计。核心算法集成了基于内部模型的 Smith 预估器以补偿滞后，
    % 并引入了动态软死区补偿（Soft Deadzone Compensation）、抗积分饱和（Anti-windup）
    % 以及软件误差死区（Software Error Deadband）机制，以解决响应迟滞和极限环震荡（Limit Cycle Oscillation）问题。
    %
    % 系统特性描述 (System Characterization):
    % 1. 通道 Q31 (过阻尼 Over-damped):
    %    - 特性：大惯性，响应迟钝，存在显著静摩擦。
    %    - 问题：起步困难，稳态易受死区补偿过度影响产生等幅震荡。
    %    - 策略：采用高增益 Smith-PI 进行快速驱动，结合带锁存功能的软死区补偿，以及较宽的误差死区来抑制稳态打桩效应。
    %
    % 2. 通道 Q32 (欠阻尼 Under-damped):
    %    - 特性：响应灵敏，阻尼比小，易超调。
    %    - 问题：系统本身接近临界稳定，易诱发高频震荡和极限环。
    %    - 策略：采用低增益控制，配合强效的软件误差死区，在稳态时切断积分作用，消除震荡源。
    %
    % 输入变量定义 (Input Variables):
    %   Q31Ref, Q32Ref : 流量设定值 (Reference Setpoint) [kg/h]
    %   Q31Real, Q32Real: 流量过程变量 (Process Variable) [kg/h]
    %   P30            : 上游压力 (Upstream Pressure) [kPa]
    %   T30            : 上游温度 (Upstream Temperature) [degC]
    %   [模型参数]      : K(静态增益), Tau(纯滞后), X_num/den(阀门传递函数系数), Tp(时间常数)
    %
    % 输出变量定义 (Output Variables):
    %   V31, V32       : 阀门控制指令 (Control Variable) [0-100%]

    % === 1. 状态记忆区 (Persistent State Memory) ===
    % 用于离散时间控制系统的状态保持
    
    persistent integrator_31 integrator_32  % PI控制器积分项累加器
    persistent model_31 model_32            % 内部快速模型状态向量 [阀位 x1; 阀速 x2; 流量 x3]
    persistent delay_buffer_31 delay_buffer_32 % 环形缓冲区，用于模拟纯滞后 Tau
    persistent head_31 head_32              % 环形缓冲区写指针
    persistent u_prev_31 u_prev_32          % 上一控制周期的输出指令 (用于差分计算)
    persistent first_run                    % 初始化标志位
    
    MAX_BUF = 1000; % 缓冲区最大长度 (支持的最大滞后步数)

    % === 系统初始化 (System Initialization) ===
    if isempty(first_run)
        integrator_31 = 0; integrator_32 = 0;
        model_31 = [0;0;0]; model_32 = [0;0;0];
        delay_buffer_31 = zeros(MAX_BUF, 1);
        delay_buffer_32 = zeros(MAX_BUF, 1);
        head_31 = 1; head_32 = 1;
        u_prev_31 = 0; u_prev_32 = 0;
        first_run = 0;
    end

    % === 2. 全局参数设定 (Global Parameters) ===
    Ts = 0.01; % 采样周期 (Sample Time) [s]
    
    % 增益调度因子计算 (Gain Scheduling Factor)
    % 依据流体力学原理，流量与压差平方根成正比。通过 Ratio 归一化过程增益，
    % 使得控制器在不同工况下保持一致的环路增益。
    Ratio = CalculateFlowRatio(P30, T30, P_ref, T_ref, R_gas, Patm);

    % ==========================================================
    %       控制策略配置 (CONTROL STRATEGY CONFIGURATION)
    % ==========================================================

    % --- 通道 31 配置 (针对过阻尼系统) ---
    % 策略逻辑：
    % 1. Kp_31 (1.8): 设置较高比例增益。Smith 预估器消除了滞后导致的相位滞后，允许提高带宽以克服过阻尼系统的惯性。
    % 2. Ti_31 (2.5): 增大积分时间常数。减弱积分作用，防止积分器在死区边缘过度充能，导致系统在目标值附近反复超调。
    % 3. Gap_31 (1.4): 适中的死区补偿值。用于在指令变化时提供额外的“启动脉冲”，克服静摩擦力。
    % 4. Err_Band_31 (0.6): 较宽的误差死区。这是消除稳态等幅震荡（Limit Cycle）的关键。当误差进入此范围，控制器停止调节，避免微小扰动触发死区补偿。
    Kp_31 = 1.8;  
    Ti_31 = 25;  
    Gap_31 = 1.4; 
    Err_Band_31 = 0.6; 

    % --- 通道 32 配置 (针对欠阻尼系统) ---
    % 策略逻辑：
    % 1. Kp_32 (0.3): 设置较低比例增益。欠阻尼系统对激励敏感，高增益极易激发系统固有频率震荡。
    % 2. Ti_32 (5.0): 极大的积分时间常数。微弱的积分作用仅用于消除长期静差，防止诱发过冲。
    % 3. Gap_32 (0.6): 较小的死区补偿。欠阻尼系统惯性小，无需强力启动，过大补偿会导致响应过激。
    % 4. Err_Band_32 (0.8): 宽误差死区。欠阻尼系统难以精确稳定在零误差，宽死区相当于提供一个“稳定停泊区”，切断极限环。
    Kp_32 = 0.3;  
    Ti_32 = 8.0;  
    Gap_32 = 0.6; 
    Err_Band_32 = 0.1; 

    % ==========================================================

    % --- 自适应控制参数计算 (Adaptive Parameter Calculation) ---
    % 根据当前的物理工况 (Ratio) 实时调整 PI 参数
    Ki_31 = Kp_31 / Ti_31;
    Kp_31_adpt = Kp_31 / Ratio;
    Ki_31_adpt = Ki_31 / Ratio;
    
    Ki_32 = Kp_32 / Ti_32;
    Kp_32_adpt = Kp_32 / Ratio;
    Ki_32_adpt = Ki_32 / Ratio;

    % ==========================================================
    %       通道 31 控制回路执行 (Control Loop Execution - Ch31)
    % ==========================================================
    
    % 1. Smith 预估器模型更新
    % 这里的模型不包含纯滞后，用于预测当前的“虚拟”无滞后响应。
    [model_31, Y_fast_31] = UpdateFastModel(model_31, u_prev_31, X31_num, X31_den, K31, Ratio, Tp31, Ts);
    
    % 2. 滞后环节模拟
    % 将无滞后响应通过延时队列，得到模型预测的有滞后响应。
    [delay_buffer_31, head_31, Y_delayed_31] = UpdateDelayBuffer(delay_buffer_31, head_31, Y_fast_31, Tau31, Ts, MAX_BUF);
    
    % 3. 模型失配补偿 (Model Mismatch Compensation)
    % 计算真实过程与模型预测之间的偏差（包含建模误差和外部干扰）。
    pred_error_31 = Q31Real - Y_delayed_31;
    
    % 4. 构造反馈主变量 (Process Variable Construction)
    % Smith 原理：反馈信号 = 无滞后模型输出 + 模型预测误差
    % 这使得主控制器感知到的对象是一个无滞后的传递函数 G(s)。
    PV_31 = Y_fast_31 + pred_error_31;
    
    % 5. 运行高级 PI 控制算法
    [u_raw_31, integrator_31, error_31] = RunPI(Q31Ref, PV_31, integrator_31, Kp_31_adpt, Ki_31_adpt, Ts, Err_Band_31);
    
    % 6. 应用带锁存功能的软死区补偿
    % 针对 31 路，增加锁存阈值至 1.5，以平滑补偿动作。
    V31 = InverseDeadzoneComp_Soft(u_raw_31, u_prev_31, Gap_31, error_31, 1.5); 
    
    u_prev_31 = V31; % 状态更新

    % ==========================================================
    %       通道 32 控制回路执行 (Control Loop Execution - Ch32)
    % ==========================================================
    
    % 步骤同上，应用针对欠阻尼系统的参数集
    [model_32, Y_fast_32] = UpdateFastModel(model_32, u_prev_32, X32_num, X32_den, K32, Ratio, Tp32, Ts);
    [delay_buffer_32, head_32, Y_delayed_32] = UpdateDelayBuffer(delay_buffer_32, head_32, Y_fast_32, Tau32, Ts, MAX_BUF);
    
    pred_error_32 = Q32Real - Y_delayed_32;
    PV_32 = Y_fast_32 + pred_error_32;
    
    [u_raw_32, integrator_32, error_32] = RunPI(Q32Ref, PV_32, integrator_32, Kp_32_adpt, Ki_32_adpt, Ts, Err_Band_32);
    
    % 32路死区补偿：使用默认阈值 1.0
    V32 = InverseDeadzoneComp_Soft(u_raw_32, u_prev_32, Gap_32, error_32, 1.0);
    
    u_prev_32 = V32;
end

%% === 核心模块 1: 高级 PI 控制器 (Advanced PI Controller) ===
% 功能：实现比例-积分控制律，集成了抗积分饱和与误差死区功能。
function [u_out, I_new, eff_err] = RunPI(Ref, Meas, I_old, Kp, Ki, Ts, ErrDeadband)
    raw_error = Ref - Meas;
    
    % --- 软件误差死区逻辑 (Software Error Deadband Logic) ---
    % 目的：消除稳态极限环震荡。
    % 原理：当误差小于预设阈值时，强制认为系统已收敛，切断误差信号。
    if abs(raw_error) < ErrDeadband
        effective_error = 0; % 有效误差置零
        I_new = I_old;       % 积分器保持（冻结）
        u_out = I_old;       % 输出保持上一时刻积分值（此时 P 项为 0）
        eff_err = 0; 
        return; 
    else
        effective_error = raw_error;
    end
    
    % --- PI 计算 ---
    P_term = Kp * effective_error;
    I_temp = I_old + Ki * effective_error * Ts; % 预积分
    u_temp = P_term + I_temp;
    
    % --- 抗积分饱和逻辑 (Anti-windup Logic - Clamping Method) ---
    % 目的：防止执行器饱和时积分器持续累积导致退饱和滞后。
    % 逻辑：当计算输出超出物理限制时，如果误差方向未能使系统退出饱和，则冻结积分器。
    if u_temp > 100
        u_out = 100;
        if effective_error > 0, I_new = I_old; else, I_new = I_temp; end
    elseif u_temp < 0
        u_out = 0;
        if effective_error < 0, I_new = I_old; else, I_new = I_temp; end
    else
        u_out = u_temp;
        I_new = I_temp;
    end
    eff_err = effective_error;
end

%% === 核心模块 2: 软死区补偿与输出锁存 (Soft Compensation & Output Latch) ===
% 功能：补偿执行器死区特性，并引入平滑机制防止控制指令跳变震荡。
function u_final = InverseDeadzoneComp_Soft(u_cmd, u_last, gap, error, err_threshold)
    delta = u_cmd - u_last;
    
    % --- 动态补偿系数 (Dynamic Compensation Factor) ---
    % 目的：实现补偿力度的渐进式变化。
    % 算法：根据当前跟踪误差的大小线性调整补偿量。误差大时全额补偿，误差小时减弱补偿。
    alpha = min(abs(error) / err_threshold, 1.0);
    real_gap = gap * alpha;
    
    % --- 输出锁存逻辑 (Output Latch Logic) ---
    % 目的：消除微小指令变化引起的震荡。
    % 逻辑：设定噪声门限 (Noise_Threshold)。若指令增量小于此门限，视为无效抖动，
    % 强制保持上一时刻输出不变。这有效防止了补偿器在临界点频繁开关。
    Noise_Threshold = 0.02; 
    
    if abs(delta) > Noise_Threshold 
        if delta > 0
            u_final = u_cmd + real_gap; % 正向补偿
        else
            u_final = u_cmd - real_gap; % 反向补偿
        end
    else
        u_final = u_last; % 锁存输出
    end
    
    % 物理限幅
    u_final = max(0, min(100, u_final));
end

%% === 辅助模块 3: 快速模型更新 (Fast Model Update) ===
% 功能：基于离散化状态空间方程，模拟无滞后的系统动态。
function [state_new, y_flow] = UpdateFastModel(state, u_in, num, den, K, Ratio, Tp, Ts)
    wn2 = den(3); zw = den(2); K_valve = num; K_total = K * Ratio;
    x1 = state(1); x2 = state(2); x3 = state(3);
    
    % 阀门二阶动力学 (Euler 积分)
    acc = K_valve * u_in - zw * x2 - wn2 * x1;
    x2_new = x2 + acc * Ts;
    x1_new = x1 + x2 * Ts;
    
    % 管道一阶流体动力学
    dy = (K_total * x1 - x3) / max(Tp, 0.1);
    x3_new = x3 + dy * Ts;
    
    state_new = [x1_new; x2_new; x3_new];
    y_flow = x3_new;
end

%% === 辅助模块 4: 延时队列管理 (Delay Buffer Management) ===
% 功能：使用环形缓冲区实现固定步长的纯滞后模拟。
function [buffer, head_idx, y_delayed] = UpdateDelayBuffer(buffer, head, y_in, Tau, Ts, MAX_BUF)
    delay_steps = round(Tau / Ts);
    delay_steps = max(1, min(delay_steps, MAX_BUF - 1));
    buffer(head) = y_in;
    read_idx = head - delay_steps;
    if read_idx < 1, read_idx = read_idx + MAX_BUF; end
    y_delayed = buffer(read_idx);
    head_idx = head + 1;
    if head_idx > MAX_BUF, head_idx = 1; end
end

%% === 辅助模块 5: 物理增益计算 (Physical Gain Calculation) ===
% 功能：基于理想气体流动方程计算流量修正系数。
function Ratio = CalculateFlowRatio(P30, T30, P_ref, T_ref, R_gas, Patm)
    Tk_dyn = T30 + 273.15; delta_P_dyn = P30 - Patm;
    if delta_P_dyn < 0, delta_P_dyn = 0; end
    Term_Dyn = sqrt((P30 * 1000 * delta_P_dyn * 1000) / (R_gas * Tk_dyn));
    Tk_ref = T_ref + 273.15; delta_P_ref = P_ref - Patm;
    if delta_P_ref < 0, delta_P_ref = 0; end
    Term_Ref = sqrt((P_ref * 1000 * delta_P_ref * 1000) / (R_gas * Tk_ref));
    if Term_Ref < 1e-6, Ratio = 1; else, Ratio = max(Term_Dyn / Term_Ref, 0.05); end
end
